simulink model "LKARefMdl"  (R2021a)
settings: Solver=FixedStepDiscrete  StartTime=0.0  StopTime=inf  FixedStep=Ts  RelTol=1e-3
values from neighbouring files (symbols this model uses):
  PredictionHorizon = 30    [helperLKASetUp.m]
  Ts = 0.1    [helperLKASetUp.m]
libraries: simulink x2, mpcadaslib x1
settings Model: Creator=The MathWorks, Inc.  LastModifiedBy=The MathWorks, Inc.
settings SolverCC: AlgebraicLoopSolver=TrustRegion
settings DataIOCC: SaveOutput=off  SaveTime=off  ReturnWorkspaceOutputs=off
settings OptimizationCC: DefaultParameterBehavior=Inlined  UseFloatMulNetSlope=on  DefaultUnderspecifiedDataType=single  UseSpecifiedMinMax=on  InlineInvariantSignals=on  EnhancedBackFolding=on  StrengthReduction=on  PassReuseOutputArgsAs=Individual arguments  ZeroExternalMemoryAtStartup=off  ZeroInternalMemoryAtStartup=off  NoFixptDivByZeroProtection=on  EfficientFloat2IntCast=on  OptimizeBlockOrder=speed  DifferentSizesBufferReuse=on  EfficientTunableParamExpr=on
settings DebuggingCC: ParameterPrecisionLossMsg=none  ParameterTunabilityLossMsg=error  SFMachineParentedDataDiag=warning  ArithmeticOperatorsInVariantConditions=warning
settings HardwareCC: ProdLongLongMode=on
settings SFSimCC: SimUseLocalCustomCode=off  MATLABDynamicMemAlloc=off  CustomCodeUndefinedFunction=UseInterfaceOnly
settings RTWCC: SystemTargetFile=ert.tlc  TemplateMakefile=ert_default_tmf  GenerateReport=on  RTWUseLocalCustomCode=off  BuildConfiguration=Faster Runs  IncludeHyperlinkInReport=on  LaunchReport=on  TargetLang=C++  GenerateTraceInfo=on  GenerateTraceReport=on  GenerateTraceReportSl=on  GenerateTraceReportSf=on  GenerateTraceReportEml=on
settings CodeAppCC: ForceParamTrailComments=on  IgnoreCustomStorageClasses=off  OperatorAnnotations=on  SimulinkDataObjDesc=on  SFDataObjDesc=on  InsertBlockDesc=on
settings ERTTargetCC: TargetLangStandard=C++03 (ISO)  GenerateSampleERTMain=on  CombineSignalStateStructs=on  SuppressErrorStatus=on  CodeInterfacePackaging=C++ class  InlinedParameterPlacement=NonHierarchical  RootIOFormat=Structure reference  ERTCustomFileTemplate=example_file_process.tlc

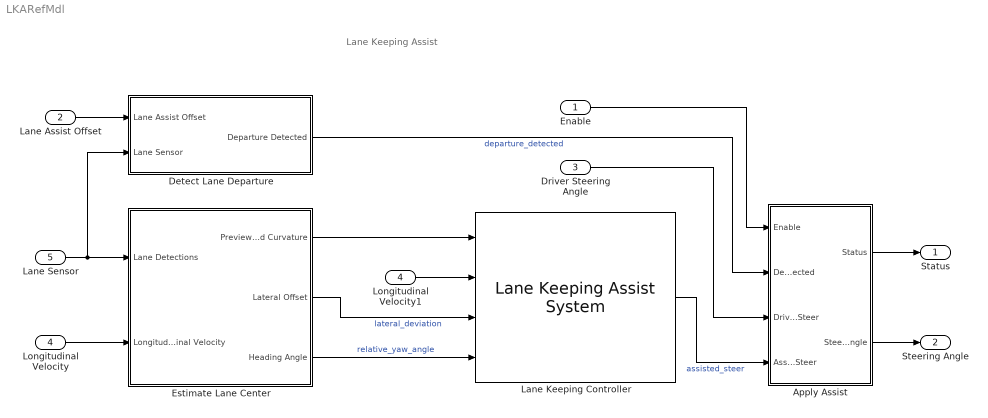
== system LKARefMdl ==
  note: Lane Keeping Assist
  Enable : Inport  OutDataTypeStr=boolean  SampleTime=Ts
  Lane Assist Offset : Inport  Port=2  OutDataTypeStr=single  Unit=m  SampleTime=Ts
  Driver Steering Angle : Inport  Port=3  Unit=rad
  Longitudinal Velocity : Inport  Port=4  OutDataTypeStr=single  Unit=m/s  SampleTime=Ts
  Lane Sensor : Inport  Port=5  OutDataTypeStr=Bus: LaneSensor  PortDimensions=[1 1]  SampleTime=Ts  BusOutputAsStruct=on
  Apply Assist : Subsystem
  Detect Lane Departure : Subsystem
  Estimate Lane Center : Subsystem  VariantControl=v2
  Lane Keeping Controller : mpcadaslib/Lane Keeping Assist System  ModelType=Use vehicle parameters  VehicleMass=m  VehicleYawInertia=Iz  LengthToFront=lf  LengthToRear=lr  FrontTireStiffness=Cf  RearTireStiffness=Cr  EgoModelMatrixA=[-4.4021 ,-12.4603;1.3913,-5.1868]  EgoModelMatrixB=[24.1270;15.8609]  EgoModelMatrixC=[1,0;0,1]  InitialLongVel=v0_ego  TransportLag=0  MinSteering=-0.5  umin_ext=off  MaxSteering=0.5  umax_ext=off  Ts=Ts  PredictionHorizon=PredictionHorizon  ControllerBehavior=0.200  suboptimal=off  maxiter=10  datatypeopt=single  optmode=off  trackmode=off
      settings: SourceProductBaseCode=MP
  Longitudinal Velocity1 : InportShadow  Port=4  OutDataTypeStr=single  Unit=m/s  SampleTime=Ts
  Status : Outport  PortDimensions=1  VectorParamsAs1DForOutWhenUnconnected=off
  Steering Angle : Outport  Port=2  PortDimensions=1  VectorParamsAs1DForOutWhenUnconnected=off
  wires:
  Longitudinal Velocity1/1 -> Lane Keeping Controller/2
  Estimate Lane Center/1(Previewed Curvature) -> Lane Keeping Controller/1
  Estimate Lane Center/2(Lateral Offset) -> Lane Keeping Controller/3  "lateral_deviation"
  Estimate Lane Center/3(Heading Angle) -> Lane Keeping Controller/4  "relative_yaw_angle"
  Lane Assist Offset/1 -> Detect Lane Departure/1(Lane Assist Offset)
  Driver Steering Angle/1 -> Apply Assist/3(Driver Steer)
  Enable/1 -> Apply Assist/1(Enable)
  Lane Keeping Controller/1 -> Apply Assist/4(Assisted Steer)  "assisted_steer"
  Apply Assist/1(Status) -> Status/1
  Apply Assist/2(Steering Angle) -> Steering Angle/1
  Detect Lane Departure/1(Departure Detected) -> Apply Assist/2(Departure Detected)  "departure_detected"
  Longitudinal Velocity/1 -> Estimate Lane Center/2(Longitudinal Velocity)
  Lane Sensor/1 -> Detect Lane Departure/2(Lane Sensor), Estimate Lane Center/1(Lane Detections)

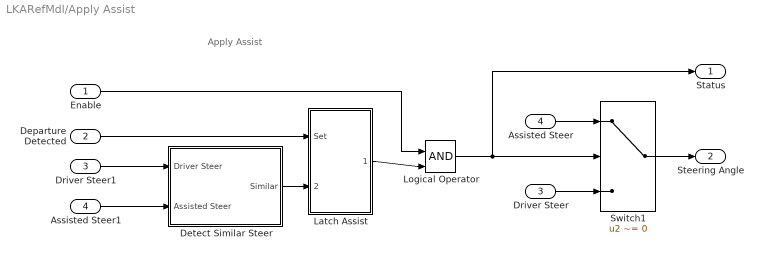
== system LKARefMdl/Apply Assist ==
  note: Apply Assist
  Enable : Inport
  Departure Detected : Inport  Port=2
  Driver Steer : Inport  Port=3
  Assisted Steer : Inport  Port=4
  Assisted Steer1 : InportShadow  Port=4
  "Detect Similar Steer " : Subsystem
  Driver Steer1 : InportShadow  Port=3
  Latch Assist : Subsystem
  Logical Operator : Logic  IconShape=distinctive  AllPortsSameDT=off  OutDataTypeStr=boolean
  Switch1 : Switch  Criteria=u2 ~= 0  Threshold=2
  Status : Outport  VectorParamsAs1DForOutWhenUnconnected=off
  Steering Angle : Outport  Port=2  Unit=rad  VectorParamsAs1DForOutWhenUnconnected=off
  wires:
  Assisted Steer/1 -> Switch1/1
  Driver Steer/1 -> Switch1/3
  Switch1/1 -> Steering Angle/1
  Enable/1 -> Logical Operator/1
  Logical Operator/1 -> Status/1, Switch1/2
  Driver Steer1/1 -> "Detect Similar Steer "/1(Driver Steer)
  Assisted Steer1/1 -> "Detect Similar Steer "/2(Assisted Steer)
  Departure Detected/1 -> Latch Assist/1(Set)
  "Detect Similar Steer "/1(Similar) -> Latch Assist/2(Reset)
  Latch Assist/1(Assist) -> Logical Operator/2

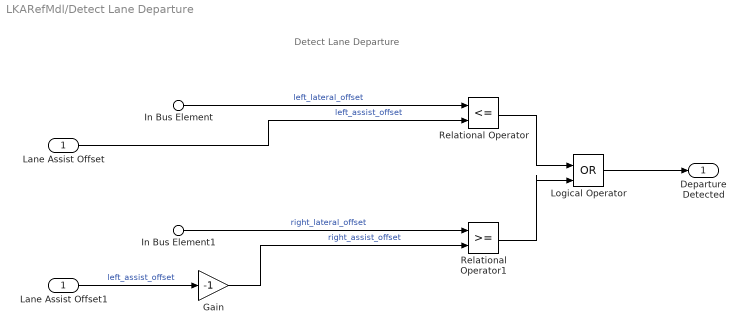
== system LKARefMdl/Detect Lane Departure ==
  note: Detect Lane Departure
  Lane Assist Offset : Inport
  In Bus Element : Inport  Port=2  PortName=Lane Sensor  Element=Left.LateralOffset
  In Bus Element1 : Inport  Port=2  PortName=Lane Sensor  Element=Right.LateralOffset
  Gain : Gain  Gain=-1
  Lane Assist Offset1 : InportShadow
  Logical Operator : Logic  Operator=OR  IconShape=distinctive  AllPortsSameDT=off  OutDataTypeStr=boolean
  Relational Operator : RelationalOperator  Operator=<=  OutDataTypeStr=boolean  RndMeth=Simplest
  Relational Operator1 : RelationalOperator  OutDataTypeStr=boolean  RndMeth=Simplest
  Departure Detected : Outport  VectorParamsAs1DForOutWhenUnconnected=off
  wires:
  Lane Assist Offset/1 -> Relational Operator/2  "left_assist_offset"
  In Bus Element/1 -> Relational Operator/1  "left_lateral_offset"
  Lane Assist Offset1/1 -> Gain/1  "left_assist_offset"
  In Bus Element1/1 -> Relational Operator1/1  "right_lateral_offset"
  Gain/1 -> Relational Operator1/2  "right_assist_offset"
  Relational Operator/1 -> Logical Operator/1
  Relational Operator1/1 -> Logical Operator/2
  Logical Operator/1 -> Departure Detected/1

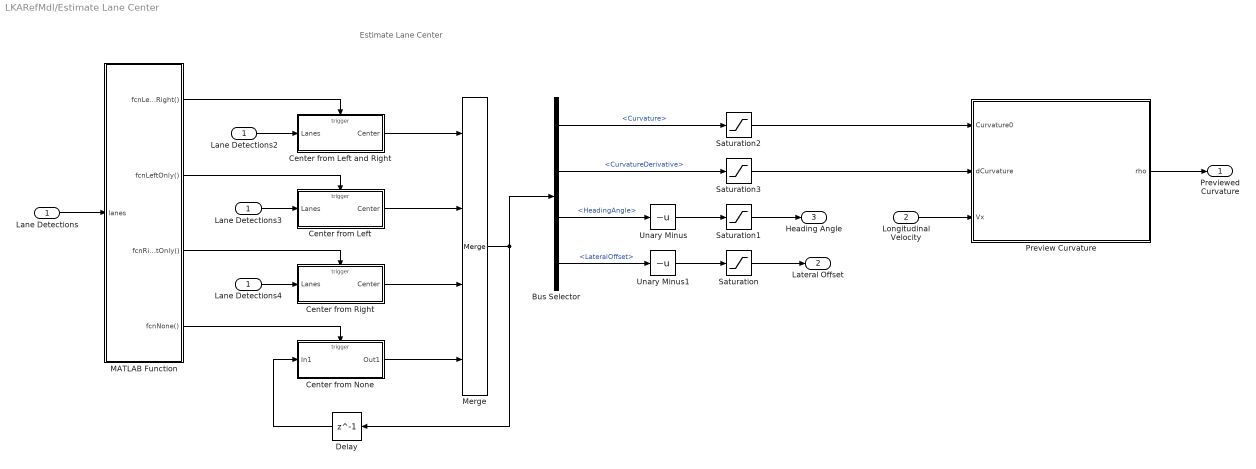
== system LKARefMdl/Estimate Lane Center ==
  note: Estimate Lane Center
  Lane Detections : Inport
  Longitudinal Velocity : Inport  Port=2  OutDataTypeStr=single
  Bus Selector : BusSelector  OutputSignals=Curvature,CurvatureDerivative,HeadingAngle,LateralOffset
  Center from Left : Subsystem  TreatAsAtomicUnit=on
  Center from Left and Right : Subsystem  TreatAsAtomicUnit=on
  Center from None : Subsystem  TreatAsAtomicUnit=on
  Center from Right : Subsystem  TreatAsAtomicUnit=on
  Delay : Delay  DelayLength=1
  Lane Detections2 : InportShadow
  Lane Detections3 : InportShadow
  Lane Detections4 : InportShadow
  MATLAB Function : MATLAB Function  TreatAsAtomicUnit=on
  Merge : Merge  Inputs=4
  Preview Curvature : MATLAB Function  TreatAsAtomicUnit=on  SystemSampleTime=Ts
  Saturation : Saturate
  Saturation1 : Saturate  UpperLimit=0.6  LowerLimit=-0.6
  Saturation2 : Saturate  UpperLimit=0.15  LowerLimit=-0.15
  Saturation3 : Saturate  UpperLimit=0.06  LowerLimit=-0.06
  Unary Minus : UnaryMinus
  Unary Minus1 : UnaryMinus
  Previewed Curvature : Outport  VectorParamsAs1DForOutWhenUnconnected=off
  Lateral Offset : Outport  Port=2  VectorParamsAs1DForOutWhenUnconnected=off
  Heading Angle : Outport  Port=3  VectorParamsAs1DForOutWhenUnconnected=off
  wires:
  Bus Selector/3 -> Unary Minus/1  "<HeadingAngle>"
  Bus Selector/4 -> Unary Minus1/1  "<LateralOffset>"
  Unary Minus1/1 -> Saturation/1
  Bus Selector/1 -> Saturation2/1  "<Curvature>"
  Bus Selector/2 -> Saturation3/1  "<CurvatureDerivative>"
  Longitudinal Velocity/1 -> Preview Curvature/3(Vx)
  Preview Curvature/1(rho) -> Previewed Curvature/1
  Unary Minus/1 -> Saturation1/1
  Saturation/1 -> Lateral Offset/1
  Saturation1/1 -> Heading Angle/1
  Saturation2/1 -> Preview Curvature/1(Curvature0)
  Saturation3/1 -> Preview Curvature/2(dCurvature)
  Merge/1 -> Delay/1, Bus Selector/1
  Center from Left/1(Center) -> Merge/2
  MATLAB Function/4(fcnNone()) -> Center from None/Trigger
  MATLAB Function/3(fcnRightOnly()) -> Center from Right/Trigger
  Lane Detections2/1 -> Center from Left and Right/1(Lanes)
  Lane Detections/1 -> MATLAB Function/1(lanes)
  Center from Left and Right/1(Center) -> Merge/1
  Delay/1 -> Center from None/1(In1)
  MATLAB Function/1(fcnLeftAndRight()) -> Center from Left and Right/Trigger
  Center from None/1(Out1) -> Merge/4
  MATLAB Function/2(fcnLeftOnly()) -> Center from Left/Trigger
  Lane Detections4/1 -> Center from Right/1(Lanes)
  Lane Detections3/1 -> Center from Left/1(Lanes)
  Center from Right/1(Center) -> Merge/3

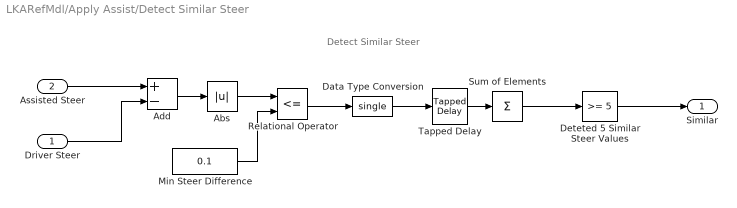
== system LKARefMdl/Apply Assist/Detect Similar Steer  ==
  note: Detect Similar Steer
  Driver Steer : Inport
  Assisted Steer : Inport  Port=2
  Abs : Abs
  Add : Sum  Inputs=+-
  Data Type Conversion : DataTypeConversion  OutDataTypeStr=single
  Deteted 5 Similar Steer Values : simulink/Logic and Bit Operations/Compare To Constant  relop=>=  const=5  OutDataTypeStr=boolean
  Min Steer Difference : Constant  Value=0.1
  Relational Operator : RelationalOperator  Operator=<=  OutDataTypeStr=boolean  RndMeth=Simplest
  Sum of Elements : Sum  Inputs=+
  Tapped Delay : simulink/Discrete/Tapped Delay  vinit=0.0  samptime=-1  NumDelays=5  DelayOrder=Oldest  includeCurrent=off
  Similar : Outport  VectorParamsAs1DForOutWhenUnconnected=off
  wires:
  Assisted Steer/1 -> Add/1
  Driver Steer/1 -> Add/2
  Add/1 -> Abs/1
  Relational Operator/1 -> Data Type Conversion/1
  Abs/1 -> Relational Operator/1
  Deteted 5 Similar Steer Values/1 -> Similar/1
  Min Steer Difference/1 -> Relational Operator/2
  Data Type Conversion/1 -> Tapped Delay/1
  Tapped Delay/1 -> Sum of Elements/1
  Sum of Elements/1 -> Deteted 5 Similar Steer Values/1

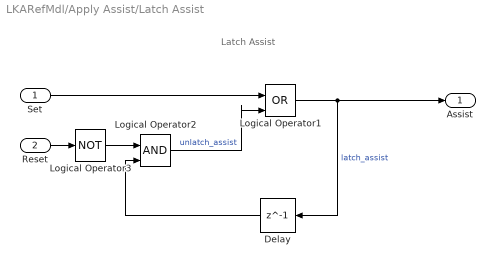
== system LKARefMdl/Apply Assist/Latch Assist ==
  note: Latch Assist
  Set : Inport
  Reset : Inport  Port=2
  Delay : Delay  DelayLength=1
  Logical Operator1 : Logic  Operator=OR  IconShape=distinctive  AllPortsSameDT=off  OutDataTypeStr=boolean
  Logical Operator2 : Logic  IconShape=distinctive  AllPortsSameDT=off  OutDataTypeStr=boolean
  Logical Operator3 : Logic  Operator=NOT  IconShape=distinctive  AllPortsSameDT=off  OutDataTypeStr=boolean
  Assist : Outport  VectorParamsAs1DForOutWhenUnconnected=off
  wires:
  Logical Operator1/1 -> Assist/1, Delay/1  "latch_assist"
  Delay/1 -> Logical Operator2/2
  Reset/1 -> Logical Operator3/1
  Logical Operator2/1 -> Logical Operator1/2  "unlatch_assist"
  Set/1 -> Logical Operator1/1
  Logical Operator3/1 -> Logical Operator2/1

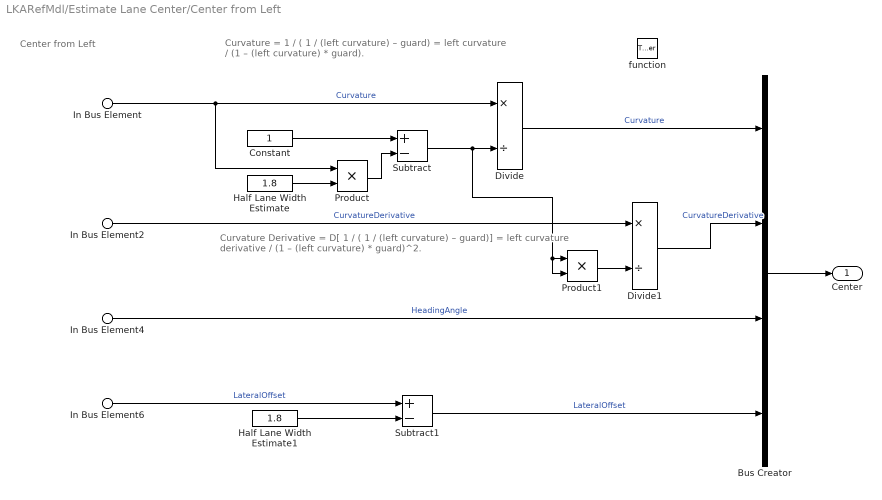
== system LKARefMdl/Estimate Lane Center/Center from Left ==
  note: Curvature
      | = 1 / ( 1 / (left curvature) – guard)
      | = left curvature / (1 – (left curvature) * guard).
  note: Center from Left
  note: Curvature Derivative
      | = D[ 1 / ( 1 / (left curvature) – guard)]
      | = left curvature derivative / (1 – (left curvature) * guard)^2.
  In Bus Element : Inport  PortName=Lanes  Element=Left.Curvature
  In Bus Element2 : Inport  PortName=Lanes  Element=Left.CurvatureDerivative
  In Bus Element4 : Inport  PortName=Lanes  Element=Left.HeadingAngle
  In Bus Element6 : Inport  PortName=Lanes  Element=Left.LateralOffset
  function : TriggerPort  TriggerType=function-call  VariantControl=Variant
  Bus Creator : BusCreator  Inputs=4
  Constant : Constant  OutDataTypeStr=Inherit: Inherit via back propagation
  Divide : Product  Inputs=*/
  Divide1 : Product  Inputs=*/
  Half Lane Width Estimate : Constant  Value=1.8  OutDataTypeStr=Inherit: Inherit via back propagation
  Half Lane Width Estimate1 : Constant  Value=1.8  OutDataTypeStr=Inherit: Inherit via back propagation
  Product : Product
  Product1 : Product
  Subtract : Sum  Inputs=+-
  Subtract1 : Sum  Inputs=+-
  Center : Outport  VectorParamsAs1DForOutWhenUnconnected=off
  wires:
  Bus Creator/1 -> Center/1
  Divide1/1 -> Bus Creator/2  "CurvatureDerivative"
  Divide/1 -> Bus Creator/1  "Curvature"
  In Bus Element4/1 -> Bus Creator/3  "HeadingAngle"
  Subtract1/1 -> Bus Creator/4  "LateralOffset"
  In Bus Element/1 -> Product/1, Divide/1  "Curvature"
  Subtract/1 -> Product1/2, Product1/1, Divide/2
  Half Lane Width Estimate/1 -> Product/2
  Constant/1 -> Subtract/1
  In Bus Element2/1 -> Divide1/1  "CurvatureDerivative"
  Product1/1 -> Divide1/2
  In Bus Element6/1 -> Subtract1/1  "LateralOffset"
  Half Lane Width Estimate1/1 -> Subtract1/2
  Product/1 -> Subtract/2

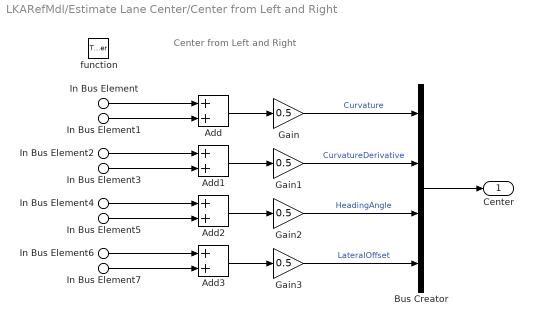
== system LKARefMdl/Estimate Lane Center/Center from Left and Right ==
  note: Center from Left and Right
  In Bus Element : Inport  PortName=Lanes  Element=Left.Curvature
  In Bus Element2 : Inport  PortName=Lanes  Element=Left.CurvatureDerivative
  In Bus Element4 : Inport  PortName=Lanes  Element=Left.HeadingAngle
  In Bus Element6 : Inport  PortName=Lanes  Element=Left.LateralOffset
  In Bus Element1 : Inport  PortName=Lanes  Element=Right.Curvature
  In Bus Element3 : Inport  PortName=Lanes  Element=Right.CurvatureDerivative
  In Bus Element5 : Inport  PortName=Lanes  Element=Right.HeadingAngle
  In Bus Element7 : Inport  PortName=Lanes  Element=Right.LateralOffset
  function : TriggerPort  TriggerType=function-call  VariantControl=Variant
  Add{,1..3} (4 alike) : Sum
  Bus Creator : BusCreator  Inputs=4
  Gain{,1..3} (4 alike) : Gain  Gain=0.5
  Center : Outport  VectorParamsAs1DForOutWhenUnconnected=off
  wires:
  Add/1 -> Gain/1
  Gain/1 -> Bus Creator/1  "Curvature"
  Add1/1 -> Gain1/1
  Gain1/1 -> Bus Creator/2  "CurvatureDerivative"
  Add2/1 -> Gain2/1
  Gain2/1 -> Bus Creator/3  "HeadingAngle"
  Add3/1 -> Gain3/1
  Gain3/1 -> Bus Creator/4  "LateralOffset"
  Bus Creator/1 -> Center/1
  In Bus Element/1 -> Add/1
  In Bus Element1/1 -> Add/2
  In Bus Element2/1 -> Add1/1
  In Bus Element3/1 -> Add1/2
  In Bus Element4/1 -> Add2/1
  In Bus Element5/1 -> Add2/2
  In Bus Element7/1 -> Add3/2
  In Bus Element6/1 -> Add3/1

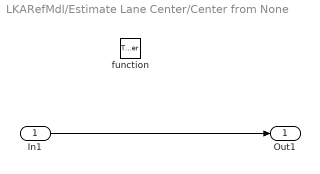
== system LKARefMdl/Estimate Lane Center/Center from None ==
  In1 : Inport
  function : TriggerPort  TriggerType=function-call  VariantControl=Variant
  Out1 : Outport  VectorParamsAs1DForOutWhenUnconnected=off
  wires:
  In1/1 -> Out1/1

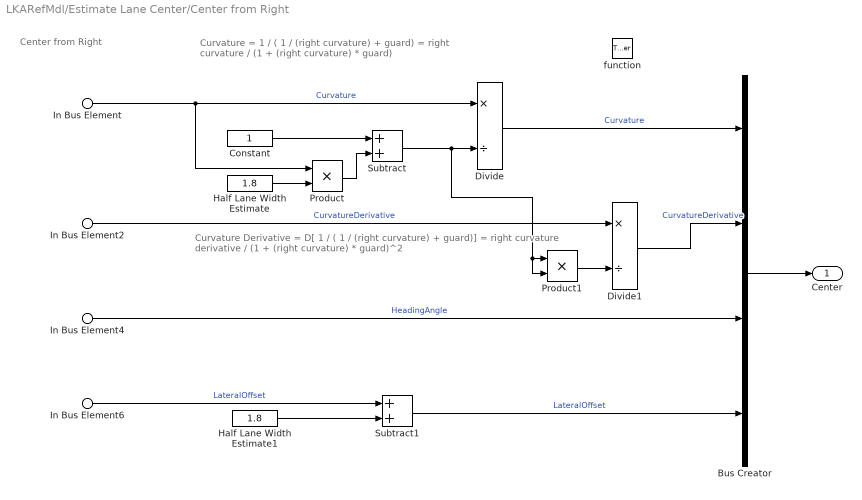
== system LKARefMdl/Estimate Lane Center/Center from Right ==
  note: Center from Right
  note: Curvature
      | = 1 / ( 1 / (right curvature) + guard)
      | = right curvature / (1 + (right curvature) * guard)
  note: Curvature Derivative
      | = D[ 1 / ( 1 / (right curvature) + guard)]
      | = right curvature derivative / (1 + (right curvature) * guard)^2
  In Bus Element : Inport  PortName=Lanes  Element=Right.Curvature
  In Bus Element2 : Inport  PortName=Lanes  Element=Right.CurvatureDerivative
  In Bus Element4 : Inport  PortName=Lanes  Element=Right.HeadingAngle
  In Bus Element6 : Inport  PortName=Lanes  Element=Right.LateralOffset
  function : TriggerPort  TriggerType=function-call  VariantControl=Variant
  Bus Creator : BusCreator  Inputs=4
  Constant : Constant  OutDataTypeStr=Inherit: Inherit via back propagation
  Divide : Product  Inputs=*/
  Divide1 : Product  Inputs=*/
  Half Lane Width Estimate : Constant  Value=1.8  OutDataTypeStr=Inherit: Inherit via back propagation
  Half Lane Width Estimate1 : Constant  Value=1.8  OutDataTypeStr=Inherit: Inherit via back propagation
  Product : Product
  Product1 : Product
  Subtract : Sum
  Subtract1 : Sum
  Center : Outport  VectorParamsAs1DForOutWhenUnconnected=off
  wires:
  In Bus Element2/1 -> Divide1/1  "CurvatureDerivative"
  Divide1/1 -> Bus Creator/2  "CurvatureDerivative"
  Product1/1 -> Divide1/2
  In Bus Element4/1 -> Bus Creator/3  "HeadingAngle"
  Half Lane Width Estimate1/1 -> Subtract1/2
  In Bus Element6/1 -> Subtract1/1  "LateralOffset"
  Divide/1 -> Bus Creator/1  "Curvature"
  Subtract1/1 -> Bus Creator/4  "LateralOffset"
  Bus Creator/1 -> Center/1
  In Bus Element/1 -> Product/1, Divide/1  "Curvature"
  Subtract/1 -> Product1/2, Product1/1, Divide/2
  Constant/1 -> Subtract/1
  Product/1 -> Subtract/2
  Half Lane Width Estimate/1 -> Product/2

== matlab function LKARefMdl/Estimate Lane Center/MATLAB Function ==
  data: lanes input
  events: fcnLeftAndRight output FUNCTION_CALL_EVENT; fcnLeftOnly output FUNCTION_CALL_EVENT; fcnRightOnly output FUNCTION_CALL_EVENT; fcnNone output FUNCTION_CALL_EVENT
function fcn(lanes)

leftStrength  = lanes.Left.Strength;
rightStrength = lanes.Right.Strength;

if (leftStrength > 0) && (rightStrength > 0)
   fcnLeftAndRight();
   
elseif leftStrength > 0
    fcnLeftOnly();
    
elseif rightStrength > 0
    fcnRightOnly();
    
else
    fcnNone();
end

== matlab function LKARefMdl/Estimate Lane Center/Preview Curvature ==
  data: rho output; Curvature0 input; dCurvature input; Vx input; Ts parameter; PredictionHorizon parameter
function rho = predictCurvature(Curvature0,dCurvature,Vx, Ts, PredictionHorizon)
% Curvature0 = initial curvature per unit length                  [1/m]
% dCurvature = (constant) derivative of curvature per unit length [1/m^2]
% CurvatureLength = length for which the clothoid model is valid [m]
% Vx = speed of vehicle

% We want to export a set of curvatures at a uniform sample time ahead.
% t is this vector which goes up to 1 second in the future or having
% enough time to reach the known length in curvature (whichever is smaller)

% To enable truncation by curvelength, mark output "rho" as varsize
%t = 0:Ts:min(1,CurvatureLength/Vx);

t = zeros(PredictionHorizon+1,1);
for i=1:numel(t)
    t(i) = (i-1).*Ts;
end

% We compute the curvature vector rho(t) using the specified clothoid model
rho = Curvature0 + dCurvature*Vx*t;
